simulink model "ex4"  (Simulink 8.7)
settings: Solver=ode45  StartTime=0.0  StopTime=10000  RelTol=1e-3
values from neighbouring files (symbols this model uses):
  M = 8    [Untitled.m]    (also in ex1.m = 4; ex10.m = 4; ex11.m = 4; ex3.m)
  SymbolRate = 1000    [ex11.m]    (also in ex2sim.m = 2; ex4sim.m = 2; ex7sim.m = 2)
libraries: commutil2 x4, commsink2 x2, commfilt2 x2, commdigbbndpm3 x2, commchan3 x1, commrandsrc2 x1
settings Model: Creator=Zhouwt  LastModifiedBy=Zhouwt
settings DataIOCC: SignalLoggingSaveFormat=ModelDataLogs
settings OptimizationCC: InitFltsAndDblsToZero=on
settings DebuggingCC: SaveWithParameterizedLinksMsg=none  SignalResolutionControl=TryResolveAllWithWarning  SolverPrmCheckMsg=warning  MultiTaskDSMMsg=warning  MultiTaskCondExecSysMsg=none  FcnCallInpInsideContextMsg=UseLocalSettings  StrictBusMsg=None
settings GRTTargetCC: TargetFcnLib=ansi_tfl_tmw.mat  GeneratePreprocessorConditionals=Use local settings  CombineOutputUpdateFcns=off  GRTInterface=on

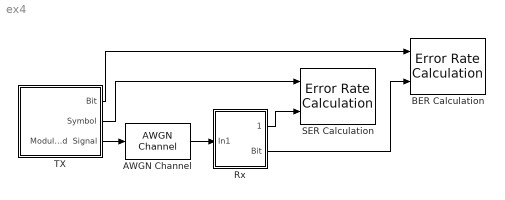
== system ex4 ==
  AWGN Channel : commchan3/AWGN Channel  InputProcessing=Inherited (this choice will be removed - see release notes)  seed=1111  noiseMode="Signal to noise ratio  (Es/No)"  EbNodB=10  EsNodB=SNR  SNRdB=10  bitsPerSym=1  Ps=1  Tsym=1/SymbolRate  variance=1
  BER Calculation : commsink2/Error Rate Calculation  N=0  st_delay=4*SymbolRate  cp_mode=Entire frame  subframe=[]  PMode=Workspace  WsName=BER  RsMode2=off  stop=off  numErr=100  maxBits=1e6
  Rx : Subsystem
  SER Calculation : commsink2/Error Rate Calculation  N=0  st_delay=SymbolRate  cp_mode=Entire frame  subframe=[]  PMode=Workspace  WsName=SER  RsMode2=off  stop=off  numErr=100  maxBits=1e6
  TX : Subsystem
  wires:
  TX/3(Modulated  Signal) -> AWGN Channel/1
  TX/2(Symbol) -> SER Calculation/1
  Rx/1(Symbol) -> SER Calculation/2
  Rx/2(Bit) -> BER Calculation/2
  TX/1(Bit) -> BER Calculation/1
  AWGN Channel/1 -> Rx/1(In1)

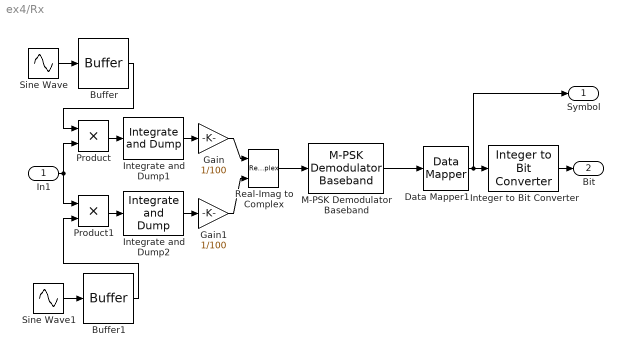
== system ex4/Rx ==
  In1 : Inport
  Buffer : Buffer  N=100*SymbolRate
  Buffer1 : Buffer  N=100*SymbolRate
  Data Mapper1 : commutil2/Data Mapper  MapMode=Gray to Binary  M=16  MapVec=[0 1 3 2 7 6 4 5]
  Gain : Gain  Gain=1/100
  Gain1 : Gain  Gain=1/100
  Integer to Bit Converter : commutil2/Integer to Bit Converter  nbits=4  signedInputValues=Unsigned  bitOrder=MSB first  outDtype=Same as input
  Integrate and Dump1 : commfilt2/Integrate and Dump  obssamples=100  offsetsamples=0  nodump=off  roundingMode=Floor  overflowMode=off  outputDataTypeStr=Inherit: Same as accumulator  outputLastDataTypeStr=Inherit: Same as accumulator
  Integrate and Dump2 : commfilt2/Integrate and Dump  obssamples=100  offsetsamples=0  nodump=off  roundingMode=Floor  overflowMode=off  outputDataTypeStr=Inherit: Same as accumulator  outputLastDataTypeStr=Inherit: Same as accumulator
  M-PSK Demodulator Baseband : commdigbbndpm3/M-PSK Demodulator Baseband  M=M  OutType=Integer  DecType=Hard decision  VarSource=Dialog  Variance=1  Dec=Gray  Mapping=[0:7]  Ph=pi/M  outDtype1=Inherit via internal rule  outDtype2=Inherit via internal rule  derotateFactorWordLen=16  derotateFactorDataTypeStr=Inherit: Same word length as input  derotateFactorLastDataTypeStr=Inherit: Same word length as input
  Product : Product  OutDataTypeStr=double  RndMeth=Zero
  Product1 : Product  OutDataTypeStr=double  RndMeth=Zero
  Real-Imag to Complex : RealImagToComplex
  Sine Wave : Sin  Amplitude=sqrt(2)  Frequency=2*pi*SymbolRate  Phase=pi/2  Samples=100  SampleTime=1/(100*SymbolRate)
  Sine Wave1 : Sin  Amplitude=sqrt(2)  Frequency=2*pi*SymbolRate  Phase=pi  Samples=100  SampleTime=1/(100*SymbolRate)
  Symbol : Outport
  Bit : Outport  Port=2
  wires:
  Integer to Bit Converter/1 -> Bit/1
  Integrate and Dump1/1 -> Gain/1
  Gain/1 -> Real-Imag to Complex/1
  Product/1 -> Integrate and Dump1/1
  Sine Wave/1 -> Buffer/1
  Buffer/1 -> Product/1
  Sine Wave1/1 -> Buffer1/1
  Buffer1/1 -> Product1/2
  Integrate and Dump2/1 -> Gain1/1
  Gain1/1 -> Real-Imag to Complex/2
  Product1/1 -> Integrate and Dump2/1
  Data Mapper1/1 -> Symbol/1, Integer to Bit Converter/1
  In1/1 -> Product/2, Product1/1
  Real-Imag to Complex/1 -> M-PSK Demodulator Baseband/1
  M-PSK Demodulator Baseband/1 -> Data Mapper1/1

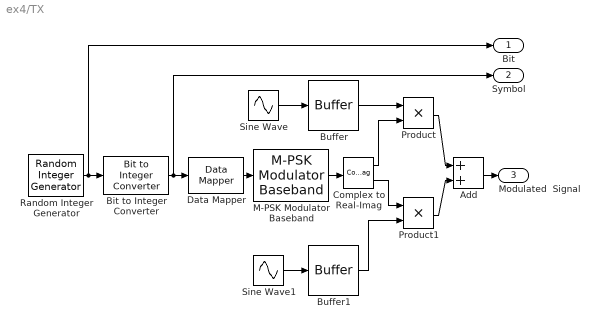
== system ex4/TX ==
  Add : Sum
  Bit to Integer Converter : commutil2/Bit to Integer Converter  nbits=4  bitOrder=MSB first  signedOutputValues=Unsigned  outDtype=Same as input  outDtypeSigned=Inherit via internal rule
  Buffer : Buffer  N=100*SymbolRate
  Buffer1 : Buffer  N=100*SymbolRate
  Complex to Real-Imag : ComplexToRealImag
  Data Mapper : commutil2/Data Mapper  MapMode=Binary to Gray  M=16  MapVec=[0 1 3 2 7 6 4 5]
  M-PSK Modulator Baseband : commdigbbndpm3/M-PSK Modulator Baseband  M=M  InType=Integer  Enc=Gray  Mapping=[0:7]  Ph=pi/M  outDtype=double  outWordLen=16  outUDDataType=sfix(16)  outFracLenMode=Best precision  outFracLen=15  outDataTypeStr=double  outLastDataTypeStr=double
  Product : Product  RndMeth=Zero
  Product1 : Product  RndMeth=Zero
  Random Integer Generator : commrandsrc2/Random Integer Generator  mul=2  seed=37  Ts=1/(4*SymbolRate)  frameBased=on  sampPerFrame=4*SymbolRate  orient=off  outDataType=double
  Sine Wave : Sin  Amplitude=sqrt(2)  Frequency=2*pi*SymbolRate  Phase=pi/2  Samples=100  SampleTime=1/(100*SymbolRate)
  Sine Wave1 : Sin  Amplitude=sqrt(2)  Frequency=2*pi*SymbolRate  Phase=pi  Samples=100  SampleTime=1/(100*SymbolRate)
  Bit : Outport
  Symbol : Outport  Port=2
  Modulated  Signal : Outport  Port=3
  wires:
  Complex to Real-Imag/1 -> Product/2
  Sine Wave/1 -> Buffer/1
  Buffer/1 -> Product/1
  Sine Wave1/1 -> Buffer1/1
  Buffer1/1 -> Product1/2
  Complex to Real-Imag/2 -> Product1/1
  Product/1 -> Add/1
  Product1/1 -> Add/2
  Add/1 -> Modulated  Signal/1
  Random Integer Generator/1 -> Bit to Integer Converter/1, Bit/1
  Bit to Integer Converter/1 -> Data Mapper/1, Symbol/1
  Data Mapper/1 -> M-PSK Modulator Baseband/1
  M-PSK Modulator Baseband/1 -> Complex to Real-Imag/1
